simulink model "IIAFS"  (R2024b)
settings: Solver=FixedStepAuto  StartTime=0.0  StopTime=80  RelTol=1e-3
libraries: simulink x4, SignalEditorBlockLib x2
settings Model: Creator=furka  LastModifiedBy=furka

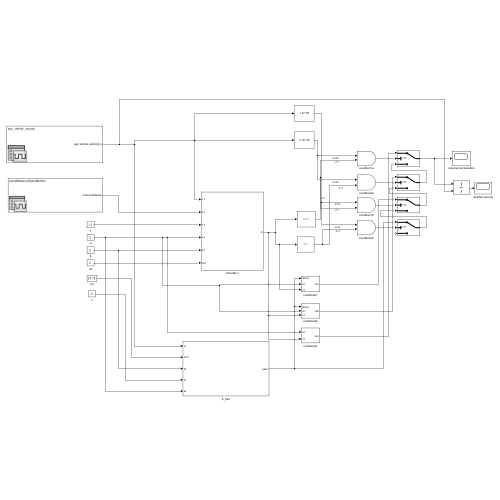
[thumbnail: Simulink's stored preview of the top-level diagram]
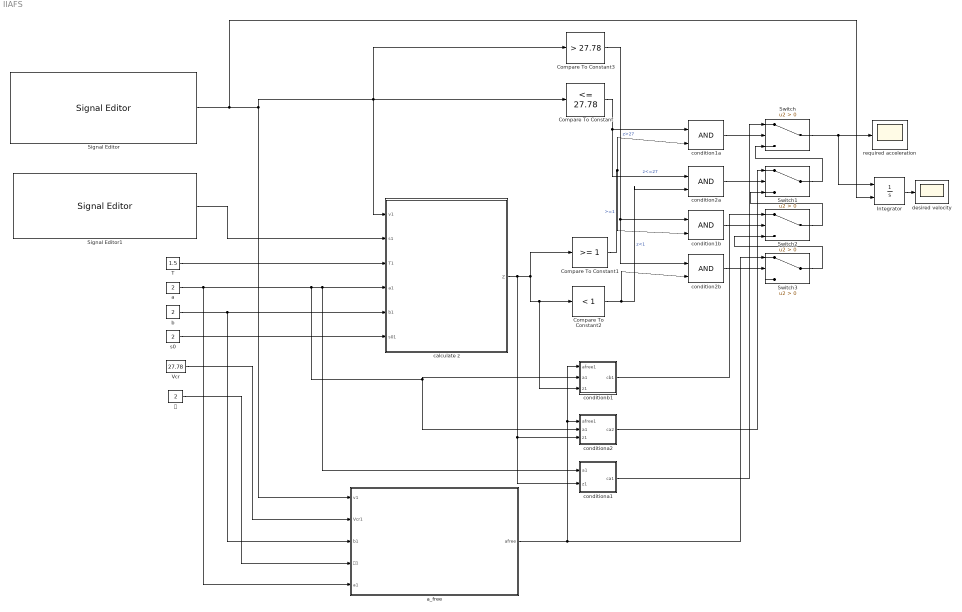
== system IIAFS ==
  Compare To Constant : simulink/Logic and Bit Operations/Compare To Constant  relop=<=  const=27.78  OutDataTypeStr=boolean
  Compare To Constant1 : simulink/Logic and Bit Operations/Compare To Constant  relop=>=  const=1  OutDataTypeStr=boolean
  Compare To Constant2 : simulink/Logic and Bit Operations/Compare To Constant  relop=<  const=1  OutDataTypeStr=boolean
  Compare To Constant3 : simulink/Logic and Bit Operations/Compare To Constant  relop=>  const=27.78  OutDataTypeStr=boolean
  Integrator : Integrator  InitialConditionSource=external  InitialCondition=0.001  IgnoreLimit=on  ZeroCross=off
  Signal Editor : SignalEditorBlockLib/Signal Editor  FileName=EGO_vehicle_velocity_Signal_Builder.mat  ActiveScenario=ego_vehicle_velocity  ActiveSignal=ego vehicle velocity(v)  IsBus=off  OutputBusObjectStr=Bus: BusObject  SampleTime=0  Interpolate=off  ZeroCross=off  OutputAfterFinalValue=Setting to zero  Unit=inherit  PreserveSignalName=on  ApplySigPropsToAllScenarios=on  ApplySigPropsToAllSignals=off
  Signal Editor1 : SignalEditorBlockLib/Signal Editor  FileName=Actual_Distance_Signal_Builder.mat  ActiveScenario=actualDistanceSignalBuilder  ActiveSignal=actual distance  IsBus=off  OutputBusObjectStr=Bus: BusObject  SampleTime=0  Interpolate=off  ZeroCross=off  OutputAfterFinalValue=Setting to zero  Unit=inherit  PreserveSignalName=on  ApplySigPropsToAllScenarios=on  ApplySigPropsToAllSignals=off
  Switch{,1..3} (4 alike) : Switch  Criteria=u2 > Threshold  SaturateOnIntegerOverflow=off  InputSameDT=off
  T : Constant  Value=1.5
  Vcr : Constant  Value=27.78
  a : Constant  Value=2
  a_free : Subsystem
  b : Constant  Value=2
  calculate z : Subsystem
  condition1a : Logic  IconShape=distinctive  AllPortsSameDT=off  OutDataTypeStr=boolean
  condition1b : Logic  IconShape=distinctive  AllPortsSameDT=off  OutDataTypeStr=boolean
  condition2a : Logic  IconShape=distinctive  AllPortsSameDT=off  OutDataTypeStr=boolean
  condition2b : Logic  IconShape=distinctive  AllPortsSameDT=off  OutDataTypeStr=boolean
  conditiona1 : Subsystem
  conditiona2 : Subsystem
  conditionb1 : Subsystem
  desired velocity : Scope
  required acceleration : Scope
  s0 : Constant  Value=2
  𝛿 : Constant  Value=2
  wires:
  Signal Editor/1 -> Integrator/2, Compare To Constant3/1, Compare To Constant/1, calculate z/1(v1), a_free/1(v1)
  T/1 -> calculate z/3(T1)
  b/1 -> a_free/3(b1), calculate z/5(b1)
  a/1 -> conditiona1/1(a1), calculate z/4(a1), conditiona2/2(a1), conditionb1/2(a1), a_free/5(a1)
  s0/1 -> calculate z/6(s01)
  Signal Editor1/1 -> calculate z/2(s1)
  calculate z/1(Z) -> conditiona1/2(z1), conditiona2/3(z1), Compare To Constant2/1, conditionb1/3(z1), Compare To Constant1/1
  Compare To Constant/1 -> condition2a/1, condition1a/1  "z<=27"
  Compare To Constant1/1 -> condition1a/2, condition1b/2  ">=1"
  Compare To Constant2/1 -> condition2b/2, condition2a/2  "z<1"
  Vcr/1 -> a_free/2(Vcr1)
  𝛿/1 -> a_free/4(𝛿1)
  a_free/1(afree) -> conditiona2/1(afree1), conditionb1/1(afree1), Switch3/1
  Compare To Constant3/1 -> condition2b/1, condition1b/1  "z>27"
  condition1a/1 -> Switch/2
  conditiona1/1(ca1) -> Switch/1
  condition2a/1 -> Switch1/2
  conditiona2/1(ca2) -> Switch1/1
  condition1b/1 -> Switch2/2
  conditionb1/1(cb1) -> Switch2/1
  condition2b/1 -> Switch3/2
  Switch1/1 -> Switch/3
  Switch2/1 -> Switch1/3
  Switch3/1 -> Switch2/3
  Switch/1 -> Integrator/1, required acceleration/1
  Integrator/1 -> desired velocity/1

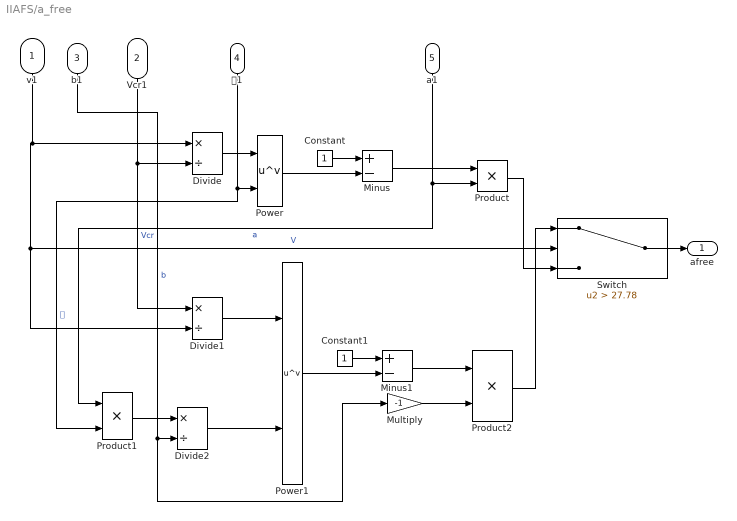
== system IIAFS/a_free ==
  v1 : Inport
  Vcr1 : Inport  Port=2
  b1 : Inport  Port=3
  𝛿1 : Inport  Port=4
  a1 : Inport  Port=5
  Constant : Constant
  Constant1 : Constant
  Divide : Product  Inputs=*/
  Divide1 : Product  Inputs=*/
  Divide2 : Product  Inputs=*/
  Minus : Sum  Inputs=+-
  Minus1 : Sum  Inputs=+-
  Multiply : Gain  Gain=-1
  Power : Math  Operator=pow
  Power1 : Math  Operator=pow
  Product : Product
  Product1 : Product
  Product2 : Product
  Switch : Switch  Criteria=u2 > Threshold  Threshold=27.78  SaturateOnIntegerOverflow=off  InputSameDT=off
  afree : Outport
  wires:
  Vcr1/1 -> Divide/2, Divide1/1  "Vcr"
  Divide/1 -> Power/1
  𝛿1/1 -> Product1/2, Power/2  "𝛿"
  Constant/1 -> Minus/1
  Power/1 -> Minus/2
  Minus/1 -> Product/1
  a1/1 -> Product1/1, Product/2  "a"
  v1/1 -> Divide/1, Switch/2, Divide1/2  "V"
  Product/1 -> Switch/3
  Divide1/1 -> Power1/1
  Product1/1 -> Divide2/1
  b1/1 -> Divide2/2, Multiply/1  "b"
  Divide2/1 -> Power1/2
  Power1/1 -> Minus1/2
  Constant1/1 -> Minus1/1
  Minus1/1 -> Product2/1
  Multiply/1 -> Product2/2
  Switch/1 -> afree/1
  Product2/1 -> Switch/1

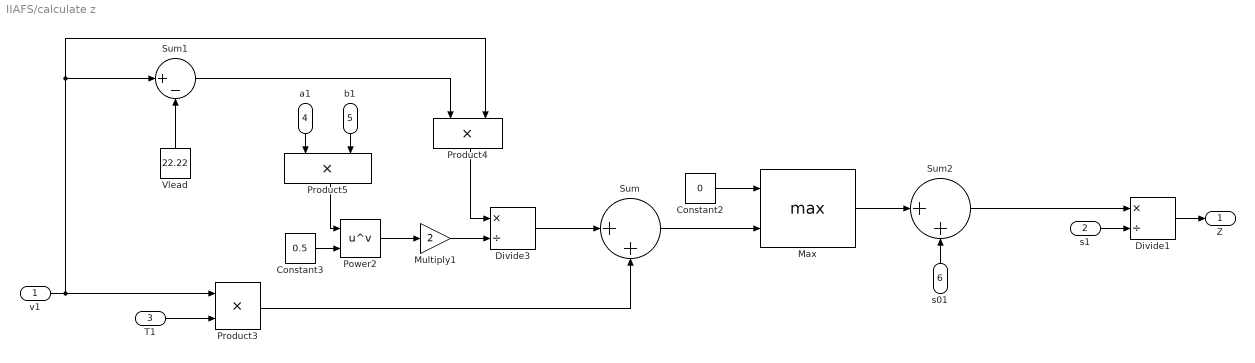
== system IIAFS/calculate z ==
  v1 : Inport
  s1 : Inport  Port=2
  T1 : Inport  Port=3
  a1 : Inport  Port=4
  b1 : Inport  Port=5
  s01 : Inport  Port=6
  Constant2 : Constant  Value=0
  Constant3 : Constant  Value=0.5
  Divide1 : Product  Inputs=*/
  Divide3 : Product  Inputs=*/
  Max : MinMax  Function=max  Inputs=2
  Multiply1 : Gain  Gain=2
  Power2 : Math  Operator=pow
  Product3 : Product
  Product4 : Product
  Product5 : Product
  Sum : Sum  Inputs=|++
  Sum1 : Sum  Inputs=|+-
  Sum2 : Sum  Inputs=|++
  Vlead : Constant  Value=22.22
  Z : Outport
  wires:
  Sum/1 -> Max/2
  T1/1 -> Product3/2
  Product3/1 -> Sum/2
  Constant2/1 -> Max/1
  Product4/1 -> Divide3/1
  Multiply1/1 -> Divide3/2
  Constant3/1 -> Power2/2
  Product5/1 -> Power2/1
  Power2/1 -> Multiply1/1
  Divide3/1 -> Sum/1
  Sum1/1 -> Product4/1
  Vlead/1 -> Sum1/2
  v1/1 -> Product3/1, Product4/2, Sum1/1
  a1/1 -> Product5/1
  b1/1 -> Product5/2
  Max/1 -> Sum2/1
  s01/1 -> Sum2/2
  Sum2/1 -> Divide1/1
  s1/1 -> Divide1/2
  Divide1/1 -> Z/1

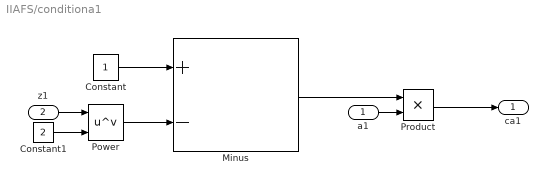
== system IIAFS/conditiona1 ==
  a1 : Inport
  z1 : Inport  Port=2
  Constant : Constant
  Constant1 : Constant  Value=2
  Minus : Sum  Inputs=+-
  Power : Math  Operator=pow
  Product : Product
  ca1 : Outport
  wires:
  Constant/1 -> Minus/1
  Constant1/1 -> Power/2
  z1/1 -> Power/1
  Power/1 -> Minus/2
  Minus/1 -> Product/1
  a1/1 -> Product/2
  Product/1 -> ca1/1

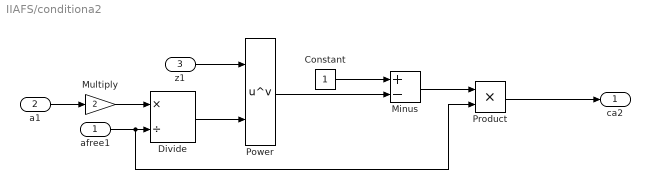
== system IIAFS/conditiona2 ==
  afree1 : Inport
  a1 : Inport  Port=2
  z1 : Inport  Port=3
  Constant : Constant
  Divide : Product  Inputs=*/
  Minus : Sum  Inputs=+-
  Multiply : Gain  Gain=2
  Power : Math  Operator=pow
  Product : Product
  ca2 : Outport
  wires:
  a1/1 -> Multiply/1
  Multiply/1 -> Divide/1
  afree1/1 -> Product/2, Divide/2
  z1/1 -> Power/1
  Divide/1 -> Power/2
  Constant/1 -> Minus/1
  Power/1 -> Minus/2
  Minus/1 -> Product/1
  Product/1 -> ca2/1

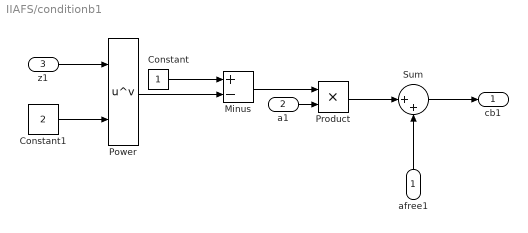
== system IIAFS/conditionb1 ==
  afree1 : Inport
  a1 : Inport  Port=2
  z1 : Inport  Port=3
  Constant : Constant
  Constant1 : Constant  Value=2
  Minus : Sum  Inputs=+-
  Power : Math  Operator=pow
  Product : Product
  Sum : Sum  Inputs=|++
  cb1 : Outport
  wires:
  afree1/1 -> Sum/2
  z1/1 -> Power/1
  Constant/1 -> Minus/1
  Power/1 -> Minus/2
  Sum/1 -> cb1/1
  Constant1/1 -> Power/2
  Minus/1 -> Product/1
  a1/1 -> Product/2
  Product/1 -> Sum/1
